simulink library "csc_egc_earth_grv_cancel_lib"  (R2014b)
settings: Solver=ode113  StartTime=0.0  StopTime=10.0  RelTol=1e-3
values from neighbouring files (symbols this model uses):
  coarse_thr_on_bias = 0.5    [csc_cac_coarse_acs_cntrl_mtv_init.m]
  force_1_to_12 = F1+F2+F3+F4+F5+F6+F7+F8+F9+F10+F11+F12    [csc_cac_coarse_acs_cntrl_mtv_init.m]
undefined symbols (not defined in the file or in its folder): csc_egc_dt, tpl_egc_throttle_to_thrust
libraries: simulink x4, util_common_lib x3, util_event_lib x2, util_info_lib x1, csu_cpt_chamber_pressure_throttle_cmd_lib x1, util_quat_lib x1
settings Model: Creator=Jim Kaidy  LastModifiedBy=tgorton

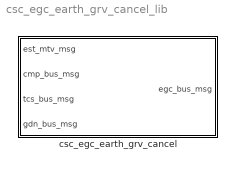
== system csc_egc_earth_grv_cancel_lib ==
  csc_egc_earth_grv_cancel : Subsystem  Tag=OFSW; MDL_TICK=TCS_BUS_MSG  TreatAsAtomicUnit=on  SystemSampleTime=csc_egc_dt

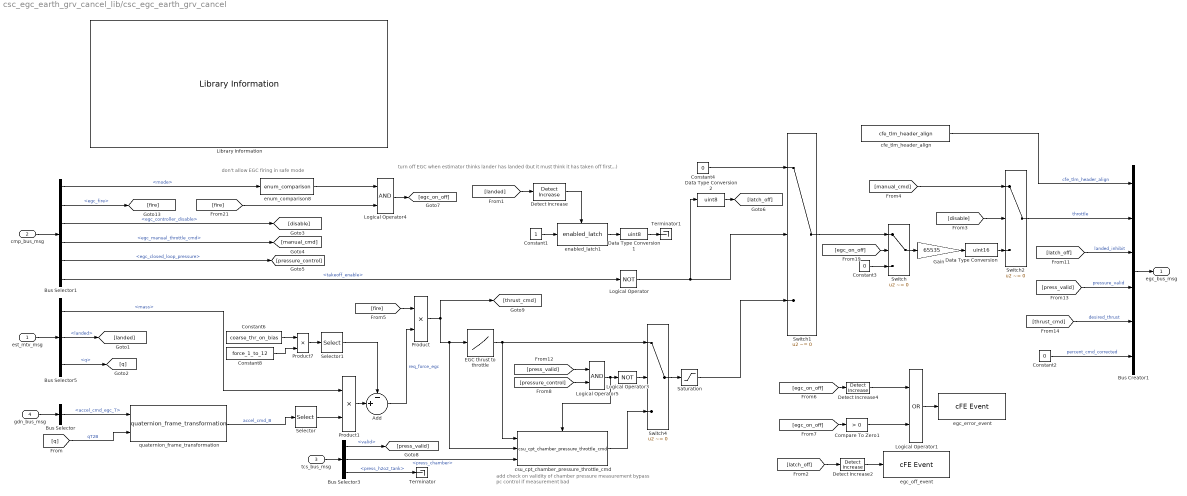
== system csc_egc_earth_grv_cancel_lib/csc_egc_earth_grv_cancel ==
  note: turn off EGC when estimator thinks lander has landed (but it must think it has taken off first...)
  note: add check on validity of chamber pressure measurement
      | bypass pc control if measurement bad
  note: don't allow EGC firing in safe mode
  est_mtv_msg : Inport  OutDataTypeStr=Bus: est_mtv_msg
  cmp_bus_msg : Inport  Port=2  OutDataTypeStr=Bus: cmp_mtv_msg
  tcs_bus_msg : Inport  Port=3  OutDataTypeStr=Bus: tcs_bus_msg
  gdn_bus_msg : Inport  Port=4  OutDataTypeStr=Bus: gdn_bus_msg
  Add : Sum  Inputs=-+|
  Bus Creator1 : BusCreator  Inputs=6  OutDataTypeStr=Bus: egc_bus_msg  NonVirtualBus=on
  Bus Selector : BusSelector  OutputSignals=accel_cmd_egc_T
  Bus Selector1 : BusSelector  OutputSignals=mode,egc_fire,egc_controller_disable,egc_manual_throttle_cmd,egc_closed_loop_pressure,takeoff_enable
  Bus Selector3 : BusSelector  OutputSignals=valid,converted_pressures.press_chamber,converted_pressures.press_h2o2_tank
  Bus Selector5 : BusSelector  OutputSignals=mass,landed,q
  Compare To Zero1 : simulink/Logic and Bit Operations/Compare To Zero  relop=>  OutDataTypeStr=boolean
  Constant1 : Constant
  Constant2 : Constant  Value=0
  Constant3 : Constant  Value=0
  Constant4 : Constant  Value=0
  Constant6 : Constant  Value=coarse_thr_on_bias
  Constant8 : Constant  Value=force_1_to_12
  Data Type Conversion : DataTypeConversion  OutDataTypeStr=uint16
  Data Type Conversion1 : DataTypeConversion  OutDataTypeStr=uint8
  Data Type Conversion2 : DataTypeConversion  OutDataTypeStr=uint8
  Detect Increase : simulink/Logic and Bit Operations/Detect Increase  vinit=1  InputProcessing=Inherited  OutDataTypeStr=boolean
  Detect Increase2 : simulink/Logic and Bit Operations/Detect Increase  vinit=0.0  InputProcessing=Inherited  OutDataTypeStr=boolean
  Detect Increase4 : simulink/Logic and Bit Operations/Detect Increase  vinit=0.0  InputProcessing=Inherited  OutDataTypeStr=boolean
  EGC thrust to throttle : Lookup  InputValues=tpl_egc_throttle_to_thrust(:,2)  Table=tpl_egc_throttle_to_thrust(:,1)  LookUpMeth=Interpolation-Use End Values
  Gain : Gain  Gain=65535
  Library Information : util_info_lib/Library Information  owner='NONE'
  Logical Operator : Logic  Operator=NOT  AllPortsSameDT=off  OutDataTypeStr=boolean
  Logical Operator1 : Logic  Operator=OR  AllPortsSameDT=off  OutDataTypeStr=boolean
  Logical Operator3 : Logic  Operator=NOT  AllPortsSameDT=off  OutDataTypeStr=boolean
  Logical Operator4 : Logic  AllPortsSameDT=off  OutDataTypeStr=boolean
  Logical Operator5 : Logic  AllPortsSameDT=off  OutDataTypeStr=boolean
  Product : Product
  Product1 : Product
  Product7 : Product
  Saturation : Saturate  UpperLimit=1.0  LowerLimit=0
      settings: AttributesFormatString=|
      | %<UpperLimit>
      | %<LowerLimit>
  Selector : Selector  InputPortWidth=3  Indices=[3]
  Selector1 : Selector  InputPortWidth=3  Indices=[3]
  Switch{,1..2,4} (4 alike) : Switch  Criteria=u2 ~= 0
  Terminator : Terminator
  Terminator1 : Terminator
  cfe_tlm_header_align : util_common_lib/cfe_tlm_header_align
  csu_cpt_chamber_pressure_throttle_cmd : csu_cpt_chamber_pressure_throttle_cmd_lib/csu_cpt_chamber_pressure_throttle_cmd
  egc_error_event : util_event_lib/cFE Event  event_message='EGC has invalid weight offset command. EGC will not fire.'  event_id=20  event_severity=ERROR  event_filtered=off  event_mask=1  event_use_enums=off  event_enum_types={}
  egc_off_event : util_event_lib/cFE Event  event_message='EGC has latched OFF based on EST landed flag.'  event_id=20  event_severity=ERROR  event_filtered=off  event_mask=1  event_use_enums=off  event_enum_types={}
  enabled_latch1 : util_common_lib/enabled_latch  initial_output=0
  enum_comparison8 : util_common_lib/enum_comparison  comparison_type=~=
  quaternion_frame_transformation : util_quat_lib/quaternion_frame_transformation  SystemSampleTime=-1
  egc_bus_msg : Outport  OutDataTypeStr=Bus: egc_bus_msg
  wires:
  Data Type Conversion2/1 -> [latch_off]
  Logical Operator/1 -> Data Type Conversion2/1, Switch1/2
  Bus Selector1/6 -> Logical Operator/1  "<takeoff_enable>"
  quaternion_frame_transformation/1 -> Selector/1  "accel_cmd_B"
  [q] -> quaternion_frame_transformation/2  "qT2B"
  Bus Selector5/3 -> [q]  "<q>"
  Selector1/1 -> Add/1
  Selector/1 -> Product1/2
  Add/1 -> Product/2  "req_force_egc"
  Product7/1 -> Selector1/1
  Constant6/1 -> Product7/1
  Constant8/1 -> Product7/2
  Product1/1 -> Add/2
  Bus Selector/1 -> quaternion_frame_transformation/1  "<accel_cmd_egc_T>"
  gdn_bus_msg/1 -> Bus Selector/1
  [fire] -> Product/1
  Bus Selector1/2 -> [fire]  "<egc_fire>"
  Logical Operator5/1 -> Logical Operator3/1, csu_cpt_chamber_pressure_throttle_cmd/Enable
  Bus Selector3/2 -> csu_cpt_chamber_pressure_throttle_cmd/3  "<press_chamber>"
  Switch4/1 -> Saturation/1
  Constant2/1 -> Bus Creator1/6  "percent_cmd_corrected"
  [thrust_cmd] -> Bus Creator1/5  "desired_thrust"
  [press_valid] -> Logical Operator5/1
  Bus Selector3/1 -> [press_valid]  "<valid>"
  enabled_latch1/1 -> Data Type Conversion1/1
  [press_valid] -> Bus Creator1/4  "pressure_valid"
  [latch_off] -> Bus Creator1/3  "landed_inhibit"
  [latch_off] -> Detect Increase2/1
  Data Type Conversion1/1 -> Terminator1/1
  Bus Selector3/3 -> Terminator/1  "<press_h2o2_tank>"
  Detect Increase2/1 -> egc_off_event/1
  Logical Operator4/1 -> [egc_on_off]
  enum_comparison8/1 -> Logical Operator4/1
  Bus Selector1/1 -> enum_comparison8/1  "<mode>"
  Logical Operator3/1 -> Switch4/2
  Bus Selector1/5 -> [pressure_control]  "<egc_closed_loop_pressure>"
  tcs_bus_msg/1 -> Bus Selector3/1
  [pressure_control] -> Logical Operator5/2
  csu_cpt_chamber_pressure_throttle_cmd/1 -> Switch4/3
  EGC thrust to throttle/1 -> Switch4/1, csu_cpt_chamber_pressure_throttle_cmd/1
  cfe_tlm_header_align/1 -> Bus Creator1/1  "cfe_tlm_header_align"
  [fire] -> Logical Operator4/2
  cmp_bus_msg/1 -> Bus Selector1/1
  Gain/1 -> Data Type Conversion/1
  Bus Creator1/1 -> egc_bus_msg/1
  Bus Selector5/1 -> Product1/1  "<mass>"
  Switch/1 -> Gain/1
  Product/1 -> [thrust_cmd], EGC thrust to throttle/1, csu_cpt_chamber_pressure_throttle_cmd/2
  est_mtv_msg/1 -> Bus Selector5/1
  Data Type Conversion/1 -> Switch2/3
  [egc_on_off] -> Switch/2
  Constant3/1 -> Switch/3
  Bus Selector5/2 -> [landed]  "<landed>"
  Switch1/1 -> Switch/1
  [landed] -> Detect Increase/1
  Detect Increase/1 -> enabled_latch1/Enable
  Constant1/1 -> enabled_latch1/1
  Constant4/1 -> Switch1/1
  Bus Selector1/3 -> [disable]  "<egc_controller_disable>"
  Bus Selector1/4 -> [manual_cmd]  "<egc_manual_throttle_cmd>"
  [disable] -> Switch2/2
  [manual_cmd] -> Switch2/1
  Switch2/1 -> Bus Creator1/2  "throttle"
  Saturation/1 -> Switch1/3
  [egc_on_off] -> Detect Increase4/1
  [egc_on_off] -> Compare To Zero1/1
  Compare To Zero1/1 -> Logical Operator1/2
  Detect Increase4/1 -> Logical Operator1/1
  Logical Operator1/1 -> egc_error_event/1
